simulink library "LIB_CycleControl"  (R2018b)
settings: Solver=VariableStepAuto  StartTime=0.0  StopTime=10.0  RelTol=1e-3
undefined symbols (not defined in the file or in its folder): eActuators, eRespiratorStates, NActuatorActive, nBlowerCmdInit, nBlowerCmdMax, nBlowerCmdMin, nBlowerDecHigh, nBlowerDecMedium, nBlowerIncHigh, nBlowerIncLow, nBlowerIncMedium, NBlowerSpeedIncCorrectionGain, NBlowerValveDerivativeGain, NBlowerValveIntegralGain, NBlowerValveIntegralHighGain, NBlowerValvePropGain, NCyclePerMinMax, NCyclePerMinMin, NMaxPressureSample, NPatientValveDerivativeGain, NPatientValveIntegralGain, NPatientValveIntegralHighGain, NPatientValvePropGain, pBlowerValveOutletOffset, pDiffMaxThdForPlateauPlausibility, pDiffThdForBlowerValveControlActivation, pDiffThdForPatientValveControlActivation, pErrorPlausibilityThd, pErrorThdForHighBlowerDec, pStaticErrorThdForHighBlowerInc, rPIDIntegralMaxTermForBlowerValve, rPIDIntegralMaxTermForPatientValve, rPIDIntegralMinTermForBlowerValve, rPIDIntegralMinTermForPatientValve, tBlowerValveOpen, tDelayBeforeRespiratorCycleStart, tDelayForRespiratorStop, tPatientValveOpen, tPhase1Ofs, tStopInhalationPhase1Min
libraries: simulink x62, simulink_need_slupdate x4, simulink_extras x3
(part 3 of 4)

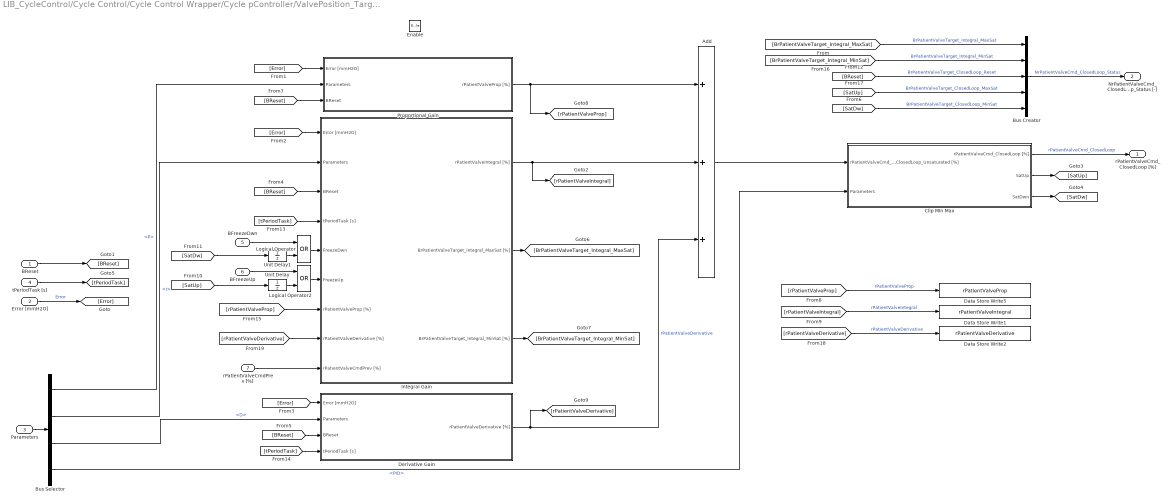
== system LIB_CycleControl/Cycle Control/Cycle Control Wrapper/Cycle pController/ValvePosition_Target/Exhalation/Patient Valve Control/PID Patient Valve ==
  BReset : Inport
  Error [mmH2O] : Inport  Port=2
  Parameters : Inport  Port=3
  tPeriodTask [s] : Inport  Port=4
  BFreezeDwn : Inport  Port=5
  BFreezeUp : Inport  Port=6
  rPatientValveCmdPrev [%] : Inport  Port=7
  Enable : EnablePort
  Add : Sum  Inputs=+++
  Bus Creator : BusCreator  Inputs=5
  Bus Selector : BusSelector  OutputSignals=P,I,D,PID
  Clip MIn Max : Subsystem
  Data Store Write1 : DataStoreWrite  DataStoreName=rPatientValveIntegral
  Data Store Write2 : DataStoreWrite  DataStoreName=rPatientValveDerivative
  Data Store Write5 : DataStoreWrite  DataStoreName=rPatientValveProp
  Derivative Gain : Subsystem
  Integral Gain : Subsystem
  Logical Operator : Logic  Operator=OR  AllPortsSameDT=off  OutDataTypeStr=boolean
  Logical Operator2 : Logic  Operator=OR  AllPortsSameDT=off  OutDataTypeStr=boolean
  Proportional Gain : Subsystem
  Unit Delay : UnitDelay  SampleTime=-1
  Unit Delay1 : UnitDelay  SampleTime=-1
  rPatientValveCmd_ClosedLoop [%] : Outport
  NrPatientValveCmd_ClosedLoop_Status [-] : Outport  Port=2
  wires:
  [rPatientValveDerivative] -> Data Store Write2/1  "rPatientValveDerivative"
  [rPatientValveIntegral] -> Data Store Write1/1  "rPatientValveIntegral"
  [rPatientValveProp] -> Data Store Write5/1  "rPatientValveProp"
  [BReset] -> Integral Gain/3(BReset)
  [rPatientValveDerivative] -> Integral Gain/8(rPatientValveDerivative [%])
  [rPatientValveProp] -> Integral Gain/7(rPatientValveProp [%])
  rPatientValveCmdPrev [%]/1 -> Integral Gain/9(rPatientValveCmdPrev [%])
  BReset/1 -> [BReset]
  [BReset] -> Derivative Gain/3(BReset)
  [BReset] -> Proportional Gain/3(BReset)
  [Error] -> Derivative Gain/1(Error [mmH2O])
  [Error] -> Integral Gain/1(Error [mmH2O])
  [Error] -> Proportional Gain/1(Error [mmH2O])
  Error [mmH2O]/1 -> [Error]  "Error"
  Clip MIn Max/1(rPatientValveCmd_ClosedLoop [%]) -> rPatientValveCmd_ClosedLoop [%]/1  "rPatientValveCmd_ClosedLoop"
  Bus Selector/4 -> Clip MIn Max/2(Parameters)  "<PID>"
  Add/1 -> Clip MIn Max/1(rPatientValveCmd_ClosedLoop_Unsaturated [%])
  Integral Gain/1(rPatientValveIntegral [%]) -> Add/2, [rPatientValveIntegral]
  Bus Selector/3 -> Derivative Gain/2(Parameters)  "<D>"
  Bus Selector/2 -> Integral Gain/2(Parameters)  "<I>"
  Bus Selector/1 -> Proportional Gain/2(Parameters)  "<P>"
  Parameters/1 -> Bus Selector/1
  [tPeriodTask] -> Integral Gain/4(tPeriodTask [s])
  Clip MIn Max/2(SatUp) -> [SatUp]
  Clip MIn Max/3(SatDwn) -> [SatDw]
  Logical Operator/1 -> Integral Gain/5(FreezeDwn)
  [SatDw] -> Unit Delay1/1
  BFreezeDwn/1 -> Logical Operator/1
  Logical Operator2/1 -> Integral Gain/6(FreezeUp)
  BFreezeUp/1 -> Logical Operator2/1
  [SatUp] -> Unit Delay/1
  Unit Delay/1 -> Logical Operator2/2
  Unit Delay1/1 -> Logical Operator/2
  tPeriodTask [s]/1 -> [tPeriodTask]
  [tPeriodTask] -> Derivative Gain/4(tPeriodTask [s])
  Integral Gain/3(BrPatientValveTarget_Integral_MinSat [%]) -> [BrPatientValveTarget_Integral_MinSat]
  Integral Gain/2(BrPatientValveTarget_Integral_MaxSat [%]) -> [BrPatientValveTarget_Integral_MaxSat]
  Bus Creator/1 -> NrPatientValveCmd_ClosedLoop_Status [-]/1  "NrPatientValveCmd_ClosedLoop_Status"
  Derivative Gain/1(rPatientValveDerivative [%]) -> Add/3, [rPatientValveDerivative]  "rPatientValveDerivative"
  Proportional Gain/1(rPatientValveProp [%]) -> Add/1, [rPatientValveProp]
  [BrPatientValveTarget_Integral_MaxSat] -> Bus Creator/1  "BrPatientValveTarget_Integral_MaxSat"
  [BrPatientValveTarget_Integral_MinSat] -> Bus Creator/2  "BrPatientValveTarget_Integral_MinSat"
  [BReset] -> Bus Creator/3  "BrPatientValveTarget_ClosedLoop_Reset"
  [SatUp] -> Bus Creator/4  "BrPatientValveTarget_ClosedLoop_MaxSat"
  [SatDw] -> Bus Creator/5  "BrPatientValveTarget_ClosedLoop_MinSat"

== system LIB_CycleControl/Cycle Control/Cycle Control Wrapper/Cycle pController/ValvePosition_Target/Exhalation/Patient Valve Control/Parameters ==
  note: 1/(2*Pi*Tau)
  Error [mmH2O] : Inport
  pBlowerValveOutletTarget [mmH2O] : Inport  Port=2
  Enable : EnablePort
  Bus Creator : BusCreator  Inputs=3
  Bus Creator1 : BusCreator  Inputs=3
  Bus Creator2 : BusCreator  Inputs=5
  Bus Creator3 : BusCreator  Inputs=5
  Bus Creator4 : BusCreator  Inputs='PidMax','PidMin'
  Constant1 : Constant  OutDataTypeStr=boolean
  Constant10 : Constant  Value=0  OutDataTypeStr=single
  Constant2 : Constant  Value=1/(2*pi*0.1)  OutDataTypeStr=single
  Constant25 : Constant  Value=100  OutDataTypeStr=single
  Constant26 : Constant  Value=-100  OutDataTypeStr=single
  Constant5 : Constant  Value=0  OutDataTypeStr=boolean
  Constant6 : Constant  Value=10  OutDataTypeStr=single
  Constant7 : Constant  Value=-10  OutDataTypeStr=single
  Constant9 : Constant  Value=100  OutDataTypeStr=single
  Gain PID Elaboration : Subsystem
  Parameters : Outport
  wires:
  pBlowerValveOutletTarget [mmH2O]/1 -> Gain PID Elaboration/2(pBlowerValveOutletTarget [mmH2O])
  Constant1/1 -> Bus Creator3/5  "Enable"
  Error [mmH2O]/1 -> Gain PID Elaboration/1(Error [mmH2O])
  Gain PID Elaboration/5(rPatientValveDerivativeGain [%/mmH2O]) -> Bus Creator2/5  "Gain"
  Constant2/1 -> Bus Creator2/4  "Freq"
  Constant5/1 -> Bus Creator2/3  "Enable"
  Constant7/1 -> Bus Creator2/2  "Min-"
  Constant6/1 -> Bus Creator2/1  "Max+"
  Constant25/1 -> Bus Creator/1  "Sat+"
  Constant26/1 -> Bus Creator/2  "Sat-"
  Gain PID Elaboration/2(rPIDIntegralMaxTermForBlowerValve [%]) -> Bus Creator1/1  "Max+"
  Gain PID Elaboration/3(rPIDIntegralMinTermForBlowerValve [%]) -> Bus Creator1/2  "Min-"
  Constant9/1 -> Bus Creator4/1  "PidMax"
  Constant10/1 -> Bus Creator4/2  "PidMin"
  Bus Creator3/1 -> Parameters/1
  Gain PID Elaboration/4(rPatientValveIntegralGain [%/mmH2O]) -> Bus Creator1/3  "Gain"
  Gain PID Elaboration/1(rPatientValveProportionalGain [%/mmH2O]) -> Bus Creator/3  "Gain"
  Bus Creator/1 -> Bus Creator3/1  "P"
  Bus Creator1/1 -> Bus Creator3/2  "I"
  Bus Creator2/1 -> Bus Creator3/3  "D"
  Bus Creator4/1 -> Bus Creator3/4  "PID"

== system LIB_CycleControl/Cycle Control/Cycle Control Wrapper/Cycle pController/ValvePosition_Target/Inhalation/Blower Valve Control/OL ==
  tPeriodTask [s] : Inport
  BExternalInit [-] : Inport  Port=2
  rBlowerValveCmdPrev [%] : Inport  Port=3
  Enable : EnablePort
  Constant1 : Constant  Value=tBlowerValveOpen  OutDataTypeStr=single
  Constant2 : Constant  Value=100  OutDataTypeStr=single
  Gain : Gain  Gain=-1
  Product : Product  Inputs=*/
  Product1 : Product  Inputs=*/
  Rate Lmiter : Subsystem  mask(Rate Limiter Dynamic){}
      mask help: Simulink:masks:RateLimiterDynamic_MD
  Switch3 : Switch  Criteria=u2 ~= 0
      settings: AttributesFormatString=%<Criteria>
  Unit Delay1 : UnitDelay  SampleTime=-1
  rBlowerValveOLCmd [%] : Outport
  wires:
  Constant1/1 -> Product1/2, Product/2
  Unit Delay1/1 -> Switch3/3
  tPeriodTask [s]/1 -> Rate Lmiter/1(tPeriodTask [s])
  BExternalInit [-]/1 -> Switch3/2
  Product1/1 -> Rate Lmiter/4(lo)
  Product/1 -> Rate Lmiter/2(up)
  rBlowerValveCmdPrev [%]/1 -> Switch3/1
  Switch3/1 -> Rate Lmiter/5(Y(k-1))
  Rate Lmiter/1(Y(k)) -> Unit Delay1/1, rBlowerValveOLCmd [%]/1
  Constant2/1 -> Gain/1, Product/1, Rate Lmiter/3(u)
  Gain/1 -> Product1/1

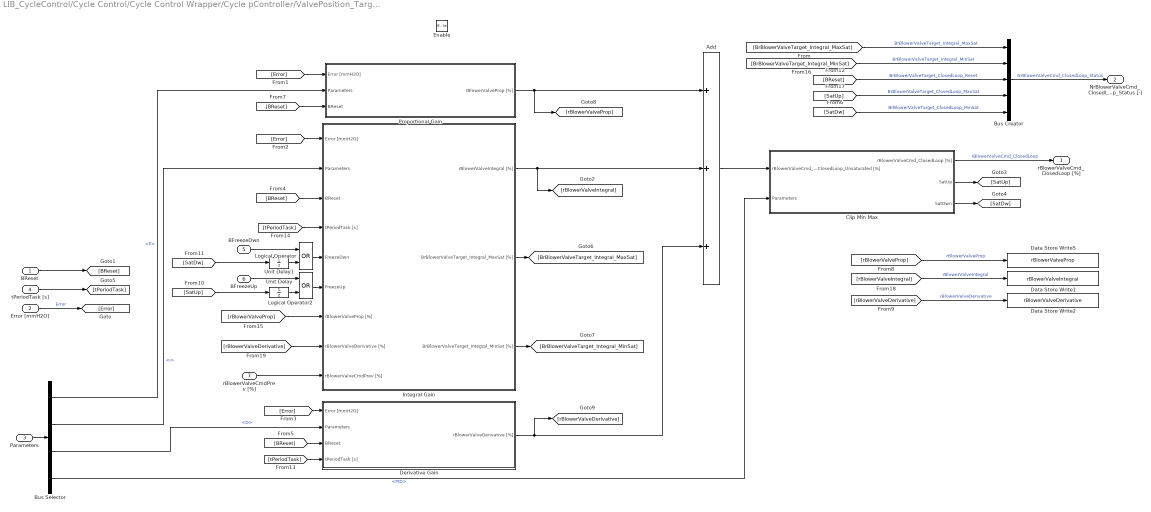
== system LIB_CycleControl/Cycle Control/Cycle Control Wrapper/Cycle pController/ValvePosition_Target/Inhalation/Blower Valve Control/PID Blower Valve ==
  BReset : Inport
  Error [mmH2O] : Inport  Port=2
  Parameters : Inport  Port=3
  tPeriodTask [s] : Inport  Port=4
  BFreezeDwn : Inport  Port=5
  BFreezeUp : Inport  Port=6
  rBlowerValveCmdPrev [%] : Inport  Port=7
  Enable : EnablePort
  Add : Sum  Inputs=+++
  Bus Creator : BusCreator  Inputs=5
  Bus Selector : BusSelector  OutputSignals=P,I,D,PID
  Clip MIn Max : Subsystem
  Data Store Write1 : DataStoreWrite  DataStoreName=rBlowerValveIntegral
  Data Store Write2 : DataStoreWrite  DataStoreName=rBlowerValveDerivative
  Data Store Write5 : DataStoreWrite  DataStoreName=rBlowerValveProp
  Derivative Gain : Subsystem
  Integral Gain : Subsystem
  Logical Operator : Logic  Operator=OR  AllPortsSameDT=off  OutDataTypeStr=boolean
  Logical Operator2 : Logic  Operator=OR  AllPortsSameDT=off  OutDataTypeStr=boolean
  Proportional Gain : Subsystem
  Unit Delay : UnitDelay  SampleTime=-1
  Unit Delay1 : UnitDelay  SampleTime=-1
  rBlowerValveCmd_ClosedLoop [%] : Outport
  NrBlowerValveCmd_ClosedLoop_Status [-] : Outport  Port=2
  wires:
  [rBlowerValveDerivative] -> Data Store Write2/1  "rBlowerValveDerivative"
  [rBlowerValveIntegral] -> Data Store Write1/1  "rBlowerValveIntegral"
  [rBlowerValveProp] -> Data Store Write5/1  "rBlowerValveProp"
  [BReset] -> Integral Gain/3(BReset)
  [rBlowerValveDerivative] -> Integral Gain/8(rBlowerValveDerivative [%])
  [rBlowerValveProp] -> Integral Gain/7(rBlowerValveProp [%])
  rBlowerValveCmdPrev [%]/1 -> Integral Gain/9(rBlowerValveCmdPrev [%])
  BReset/1 -> [BReset]
  [BReset] -> Derivative Gain/3(BReset)
  [BReset] -> Proportional Gain/3(BReset)
  [Error] -> Derivative Gain/1(Error [mmH2O])
  [Error] -> Integral Gain/1(Error [mmH2O])
  [Error] -> Proportional Gain/1(Error [mmH2O])
  Error [mmH2O]/1 -> [Error]  "Error"
  Clip MIn Max/1(rBlowerValveCmd_ClosedLoop [%]) -> rBlowerValveCmd_ClosedLoop [%]/1  "rBlowerValveCmd_ClosedLoop"
  Bus Selector/4 -> Clip MIn Max/2(Parameters)  "<PID>"
  Add/1 -> Clip MIn Max/1(rBlowerValveCmd_ClosedLoop_Unsaturated [%])
  Integral Gain/1(rBlowerValveIntegral [%]) -> Add/2, [rBlowerValveIntegral]
  Bus Selector/3 -> Derivative Gain/2(Parameters)  "<D>"
  Bus Selector/2 -> Integral Gain/2(Parameters)  "<I>"
  Bus Selector/1 -> Proportional Gain/2(Parameters)  "<P>"
  Parameters/1 -> Bus Selector/1
  [tPeriodTask] -> Integral Gain/4(tPeriodTask [s])
  Clip MIn Max/2(SatUp) -> [SatUp]
  Clip MIn Max/3(SatDwn) -> [SatDw]
  Logical Operator/1 -> Integral Gain/5(FreezeDwn)
  [SatDw] -> Unit Delay1/1
  BFreezeDwn/1 -> Logical Operator/1
  Logical Operator2/1 -> Integral Gain/6(FreezeUp)
  BFreezeUp/1 -> Logical Operator2/1
  [SatUp] -> Unit Delay/1
  Unit Delay/1 -> Logical Operator2/2
  Unit Delay1/1 -> Logical Operator/2
  tPeriodTask [s]/1 -> [tPeriodTask]
  [tPeriodTask] -> Derivative Gain/4(tPeriodTask [s])
  Integral Gain/3(BrBlowerValveTarget_Integral_MinSat [%]) -> [BrBlowerValveTarget_Integral_MinSat]
  Integral Gain/2(BrBlowerValveTarget_Integral_MaxSat [%]) -> [BrBlowerValveTarget_Integral_MaxSat]
  Bus Creator/1 -> NrBlowerValveCmd_ClosedLoop_Status [-]/1  "NrBlowerValveCmd_ClosedLoop_Status"
  Derivative Gain/1(rBlowerValveDerivative [%]) -> Add/3, [rBlowerValveDerivative]
  Proportional Gain/1(rBlowerValveProp [%]) -> Add/1, [rBlowerValveProp]
  [BrBlowerValveTarget_Integral_MaxSat] -> Bus Creator/1  "BrBlowerValveTarget_Integral_MaxSat"
  [BrBlowerValveTarget_Integral_MinSat] -> Bus Creator/2  "BrBlowerValveTarget_Integral_MinSat"
  [BReset] -> Bus Creator/3  "BrBlowerValveTarget_ClosedLoop_Reset"
  [SatUp] -> Bus Creator/4  "BrBlowerValveTarget_ClosedLoop_MaxSat"
  [SatDw] -> Bus Creator/5  "BrBlowerValveTarget_ClosedLoop_MinSat"

== system LIB_CycleControl/Cycle Control/Cycle Control Wrapper/Cycle pController/ValvePosition_Target/Inhalation/Blower Valve Control/Parameters ==
  note: 1/(2*Pi*Tau)
  Error : Inport
  Enable : EnablePort
  Bus Creator : BusCreator  Inputs=3
  Bus Creator1 : BusCreator  Inputs=3
  Bus Creator2 : BusCreator  Inputs=5
  Bus Creator3 : BusCreator  Inputs=5
  Bus Creator4 : BusCreator  Inputs='PidMax','PidMin'
  Constant1 : Constant  OutDataTypeStr=boolean
  Constant10 : Constant  Value=0  OutDataTypeStr=single
  Constant2 : Constant  Value=1/(2*pi*0.1)  OutDataTypeStr=single
  Constant25 : Constant  Value=100  OutDataTypeStr=single
  Constant26 : Constant  Value=-100  OutDataTypeStr=single
  Constant5 : Constant  Value=0  OutDataTypeStr=boolean
  Constant6 : Constant  Value=10  OutDataTypeStr=single
  Constant7 : Constant  Value=-10  OutDataTypeStr=single
  Constant9 : Constant  Value=100  OutDataTypeStr=single
  Gain PID Elaboration : Subsystem
  Parameters : Outport
  wires:
  Constant1/1 -> Bus Creator3/5  "Enable"
  Gain PID Elaboration/5(rBlowerValveDerivativeGain [%/mmH2O]) -> Bus Creator2/5  "Gain"
  Constant2/1 -> Bus Creator2/4  "Freq"
  Constant5/1 -> Bus Creator2/3  "Enable"
  Constant7/1 -> Bus Creator2/2  "Min-"
  Constant6/1 -> Bus Creator2/1  "Max+"
  Constant25/1 -> Bus Creator/1  "Sat+"
  Constant26/1 -> Bus Creator/2  "Sat-"
  Gain PID Elaboration/2(rPIDIntegralMaxTermForBlowerValve [%]) -> Bus Creator1/1  "Max+"
  Gain PID Elaboration/3(rPIDIntegralMinTermForBlowerValve [%]) -> Bus Creator1/2  "Min-"
  Constant9/1 -> Bus Creator4/1  "PidMax"
  Constant10/1 -> Bus Creator4/2  "PidMin"
  Bus Creator3/1 -> Parameters/1
  Gain PID Elaboration/4(rBlowerValveIntegralGain [%/mmH2O]) -> Bus Creator1/3  "Gain"
  Gain PID Elaboration/1(rBlowerValveProportionalGain [%/mmH2O]) -> Bus Creator/3  "Gain"
  Bus Creator/1 -> Bus Creator3/1  "P"
  Bus Creator1/1 -> Bus Creator3/2  "I"
  Bus Creator2/1 -> Bus Creator3/3  "D"
  Bus Creator4/1 -> Bus Creator3/4  "PID"
  Error/1 -> Gain PID Elaboration/1(Error)

== system LIB_CycleControl/Cycle Control/Cycle Control Wrapper/Cycle pController/ValvePosition_Target/Exhalation/Patient Valve Control/OL1/Rate Lmiter ==
  note: Y(k)
  tPeriodTask [s] : Inport
  up : Inport  Port=2
  u : Inport  Port=3
  lo : Inport  Port=4
  Y(k-1) : Inport  Port=5
  Difference Inputs1 : Sum  Description=Add in CPU  DisableCoverage=on  Inputs=+-  OutDataTypeStr=Inherit: Inherit via back propagation
  Difference Inputs2 : Sum  Description=Add in CPU  OutDataTypeStr=Inherit: Inherit via back propagation
  Saturation Dynamic : simulink/Discontinuities/Saturation Dynamic  OutMin=[]  OutMax=[]  OutDataTypeStr=Inherit: Same as second input  OutDataType=fixdt(1, 16)  OutScaling=2^-10  DoSatur=off
  delta fall limit : Product  DisableCoverage=on  Inputs=**  OutDataTypeStr=Inherit: Inherit via back propagation  SaturateOnIntegerOverflow=on
  delta rise limit : Product  DisableCoverage=on  Inputs=**  OutDataTypeStr=Inherit: Inherit via back propagation  SaturateOnIntegerOverflow=on
  Y(k) : Outport
  wires:
  Y(k-1)/1 -> Difference Inputs1/2, Difference Inputs2/2
  lo/1 -> delta fall limit/1
  u/1 -> Difference Inputs1/1
  up/1 -> delta rise limit/1
  Difference Inputs2/1 -> Y(k)/1
  delta fall limit/1 -> Saturation Dynamic/3
  delta rise limit/1 -> Saturation Dynamic/1
  Saturation Dynamic/1 -> Difference Inputs2/1
  Difference Inputs1/1 -> Saturation Dynamic/2  "( U(k) - Y(k-1) )"
  tPeriodTask [s]/1 -> delta rise limit/2, delta fall limit/2

== system LIB_CycleControl/Cycle Control/Cycle Control Wrapper/Cycle pController/ValvePosition_Target/Exhalation/Patient Valve Control/PID Patient Valve/Clip MIn Max ==
  rPatientValveCmd_ClosedLoop_Unsaturated [%] : Inport
  Parameters : Inport  Port=2
  Bus Selector : BusSelector  OutputSignals=PidMax,PidMin
  Clip1 : Subsystem  mask(PT Common Clip){}
      mask help: Input is clipped between the upper and lower limits.
      mask Help: helpview(fullfile(ptcommonroot,'help', 'clip.htm'))
  rPatientValveCmd_ClosedLoop [%] : Outport
  SatUp : Outport  Port=2
  SatDwn : Outport  Port=3
  wires:
  Clip1/2(Out) -> rPatientValveCmd_ClosedLoop [%]/1
  rPatientValveCmd_ClosedLoop_Unsaturated [%]/1 -> Clip1/2(In)
  Bus Selector/1 -> Clip1/1(Upper)  "<PidMax>"
  Parameters/1 -> Bus Selector/1
  Bus Selector/2 -> Clip1/3(Lower)  "<PidMin>"
  Clip1/1(SatUp) -> SatUp/1
  Clip1/3(SatDwn) -> SatDwn/1

== system LIB_CycleControl/Cycle Control/Cycle Control Wrapper/Cycle pController/ValvePosition_Target/Exhalation/Patient Valve Control/PID Patient Valve/Derivative Gain ==
  note: Derivative
  Error [mmH2O] : Inport
  Parameters : Inport  Port=2
  BReset : Inport  Port=3
  tPeriodTask [s] : Inport  Port=4
  Bus Selector : BusSelector  OutputSignals=Enable,Gain,Max+,Min-,Freq
  Compute Derivative : Subsystem
  rPatientValveDerivative [%] : Outport
  wires:
  [BReset] -> Compute Derivative/5(BReset)
  Bus Selector/1 -> Compute Derivative/Enable  "<Enable>"
  Bus Selector/5 -> Compute Derivative/4(Freq)  "<Freq>"
  Bus Selector/4 -> Compute Derivative/3(Min-)  "<Min->"
  Bus Selector/3 -> Compute Derivative/2(Max+)  "<Max+>"
  Bus Selector/2 -> Compute Derivative/1(Gain)  "<Gain>"
  tPeriodTask [s]/1 -> Compute Derivative/7(tPeriodTask [s])
  Error [mmH2O]/1 -> Compute Derivative/6(Error [mmH2O])
  BReset/1 -> [BReset]
  Parameters/1 -> Bus Selector/1
  Compute Derivative/1(rPatientValveDerivative [%]) -> rPatientValveDerivative [%]/1

== system LIB_CycleControl/Cycle Control/Cycle Control Wrapper/Cycle pController/ValvePosition_Target/Exhalation/Patient Valve Control/PID Patient Valve/Integral Gain ==
  Error [mmH2O] : Inport
  Parameters : Inport  Port=2
  BReset : Inport  Port=3
  tPeriodTask [s] : Inport  Port=4
  FreezeDwn : Inport  Port=5
  FreezeUp : Inport  Port=6
  rPatientValveProp [%] : Inport  Port=7
  rPatientValveDerivative [%] : Inport  Port=8
  rPatientValveCmdPrev [%] : Inport  Port=9
  Bus Selector : BusSelector  OutputSignals=Gain,Max+,Min-
  Clip : Subsystem  mask(PT Common Clip){}
      mask help: Input is clipped between the upper and lower limits.
      mask Help: helpview(fullfile(ptcommonroot,'help', 'clip.htm'))
  Init : Subsystem
  Logical Operator : Logic  AllPortsSameDT=off  OutDataTypeStr=boolean
  Logical Operator2 : Logic  Operator=NOT  AllPortsSameDT=off  OutDataTypeStr=boolean
  Logical Operator3 : Logic  AllPortsSameDT=off  OutDataTypeStr=boolean
  Logical Operator4 : Logic  Operator=NOT  AllPortsSameDT=off  OutDataTypeStr=boolean
  Product1 : Product  Inputs=3  RndMeth=Zero
  Reset? : Switch  Criteria=u2 ~= 0
  Sum1 : Sum  Inputs=|++
  Sum2 : Sum  Inputs=|++
  Unit Delay1 : UnitDelay  SampleTime=-1
  rPatientValveIntegral [%] : Outport
  BrPatientValveTarget_Integral_MaxSat [%] : Outport  Port=2
  BrPatientValveTarget_Integral_MinSat [%] : Outport  Port=3
  wires:
  Bus Selector/1 -> Product1/3  "<Gain>"
  Sum2/1 -> Reset?/1
  Init/1(Init) -> Sum2/1
  Unit Delay1/1 -> Sum1/2
  [BReset] -> Init/Enable
  BReset/1 -> [BReset]
  rPatientValveProp [%]/1 -> Init/3(rPatientValveProp [%])
  rPatientValveDerivative [%]/1 -> Init/2(rPatientValveDerivative [%])
  rPatientValveCmdPrev [%]/1 -> Init/1(rPatientValveCmdPrev [%])
  Clip/2(Out) -> Unit Delay1/1, rPatientValveIntegral [%]/1  "Error"
  Sum1/1 -> Reset?/3
  Reset?/1 -> Clip/3(In)
  Error [mmH2O]/1 -> Product1/1  "Error"
  Product1/1 -> Sum1/1, Sum2/2  "Gain*Error"
  Parameters/1 -> Bus Selector/1
  tPeriodTask [s]/1 -> Product1/2
  FreezeDwn/1 -> Logical Operator3/1
  FreezeUp/1 -> Logical Operator/1
  Clip/1(SatUp) -> BrPatientValveTarget_Integral_MaxSat [%]/1
  Clip/3(SatDwn) -> BrPatientValveTarget_Integral_MinSat [%]/1
  Bus Selector/3 -> [SatDwn]  "<Min->"
  Bus Selector/2 -> [SatUp]  "<Max+>"
  [SatUp] -> Clip/2(Upper)
  [SatDwn] -> Clip/4(Lower)
  Logical Operator/1 -> Clip/1(FreezeUp)
  Logical Operator2/1 -> Logical Operator/2
  Logical Operator3/1 -> Clip/5(FreezeDwn)
  Logical Operator4/1 -> Logical Operator3/2
  [BReset] -> Reset?/2, Logical Operator2/1, Logical Operator4/1

== system LIB_CycleControl/Cycle Control/Cycle Control Wrapper/Cycle pController/ValvePosition_Target/Exhalation/Patient Valve Control/PID Patient Valve/Proportional Gain ==
  Error [mmH2O] : Inport
  Parameters : Inport  Port=2
  BReset : Inport  Port=3
  Bus Selector : BusSelector  OutputSignals=Gain,Sat+,Sat-
  Clip : Subsystem  mask(PT Common Clip){}
      mask help: Input is clipped between the upper and lower limits.
      mask Help: helpview(fullfile(ptcommonroot,'help', 'clip.htm'))
  Constant : Constant  Value=0  OutDataTypeStr=single
  Product : Product  RndMeth=Zero
  Switch : Switch  Criteria=u2 ~= 0
  rPatientValveProp [%] : Outport
  wires:
  Parameters/1 -> Bus Selector/1
  Bus Selector/1 -> Product/1  "<Gain>"
  Switch/1 -> Product/2  "Error"
  BReset/1 -> Switch/2
  Constant/1 -> Switch/1
  Error [mmH2O]/1 -> Switch/3
  Bus Selector/2 -> Clip/1(Upper)  "<Sat+>"
  Bus Selector/3 -> Clip/3(Lower)  "<Sat->"
  Product/1 -> Clip/2(In)  "Gain*Error"
  Clip/1(Out) -> rPatientValveProp [%]/1

== system LIB_CycleControl/Cycle Control/Cycle Control Wrapper/Cycle pController/ValvePosition_Target/Exhalation/Patient Valve Control/Parameters/Gain PID Elaboration ==
  Error [mmH2O] : Inport
  pBlowerValveOutletTarget [mmH2O] : Inport  Port=2
  Compare To Zero : simulink/Logic and Bit Operations/Compare To Zero  relop=>  OutDataTypeStr=boolean
  Constant1 : Constant  Value=NPatientValveIntegralHighGain
  Constant28 : Constant  Value=NPatientValveIntegralGain
  Constant29 : Constant  Value=NPatientValveDerivativeGain
  Constant30 : Constant  Value=rPIDIntegralMaxTermForPatientValve
  Constant31 : Constant  Value=rPIDIntegralMinTermForPatientValve
  Constant32 : Constant  Value=NPatientValvePropGain
  Conv mmH2O to % : Gain  Gain=-100/1000
  Gain1 : Gain  Gain=-100/1000
  Gain2 : Gain  Gain=-100/1000
  NIntegralCorrectionPeep : Lookup_n-D  NumberOfTableDimensions=1  BreakpointsForDimension1=[0 50 100 150 200]  IndexSearchMethod=Linear search  BeginIndexSearchUsingPreviousIndexResult=on  Table=[1.5 1.5 1 0.5 0.5]  ExtrapMethod=Clip  UseLastTableValue=on  InternalRulePriority=Speed  RndMeth=Simplest  InputSameDT=on
  NPropCorrectionPeep : Lookup_n-D  NumberOfTableDimensions=1  BreakpointsForDimension1=[0 50 100 150 200]  IndexSearchMethod=Linear search  BeginIndexSearchUsingPreviousIndexResult=on  Table=[1 1 1 1 1]  ExtrapMethod=Clip  UseLastTableValue=on  InternalRulePriority=Speed  RndMeth=Simplest  InputSameDT=on
  Product : Product
  Product1 : Product
  Switch7 : Switch  Criteria=u2 ~= 0
      settings: AttributesFormatString=%<Criteria>
  rPatientValveProportionalGain [%/mmH2O] : Outport
  rPIDIntegralMaxTermForBlowerValve [%] : Outport  Port=2
  rPIDIntegralMinTermForBlowerValve [%] : Outport  Port=3
  rPatientValveIntegralGain [%/mmH2O] : Outport  Port=4
  rPatientValveDerivativeGain [%/mmH2O] : Outport  Port=5
  wires:
  Product1/1 -> Gain1/1
  NIntegralCorrectionPeep/1 -> Product1/1
  Switch7/1 -> Product1/2
  Error [mmH2O]/1 -> Compare To Zero/1
  Constant1/1 -> Switch7/1
  NPropCorrectionPeep/1 -> Product/2
  Constant32/1 -> Product/1
  Compare To Zero/1 -> Switch7/2
  Constant28/1 -> Switch7/3
  pBlowerValveOutletTarget [mmH2O]/1 -> NPropCorrectionPeep/1, NIntegralCorrectionPeep/1
  Constant31/1 -> rPIDIntegralMinTermForBlowerValve [%]/1
  Constant30/1 -> rPIDIntegralMaxTermForBlowerValve [%]/1
  Constant29/1 -> Gain2/1
  Product/1 -> Conv mmH2O to %/1
  Gain2/1 -> rPatientValveDerivativeGain [%/mmH2O]/1
  Conv mmH2O to %/1 -> rPatientValveProportionalGain [%/mmH2O]/1
  Gain1/1 -> rPatientValveIntegralGain [%/mmH2O]/1

== system LIB_CycleControl/Cycle Control/Cycle Control Wrapper/Cycle pController/ValvePosition_Target/Inhalation/Blower Valve Control/OL/Rate Lmiter ==
  note: Y(k)
  tPeriodTask [s] : Inport
  up : Inport  Port=2
  u : Inport  Port=3
  lo : Inport  Port=4
  Y(k-1) : Inport  Port=5
  Difference Inputs1 : Sum  Description=Add in CPU  DisableCoverage=on  Inputs=+-  OutDataTypeStr=Inherit: Inherit via back propagation
  Difference Inputs2 : Sum  Description=Add in CPU  OutDataTypeStr=Inherit: Inherit via back propagation
  Saturation Dynamic : simulink/Discontinuities/Saturation Dynamic  OutMin=[]  OutMax=[]  OutDataTypeStr=Inherit: Same as second input  OutDataType=fixdt(1, 16)  OutScaling=2^-10  DoSatur=off
  delta fall limit : Product  DisableCoverage=on  Inputs=**  OutDataTypeStr=Inherit: Inherit via back propagation  SaturateOnIntegerOverflow=on
  delta rise limit : Product  DisableCoverage=on  Inputs=**  OutDataTypeStr=Inherit: Inherit via back propagation  SaturateOnIntegerOverflow=on
  Y(k) : Outport
  wires:
  Y(k-1)/1 -> Difference Inputs1/2, Difference Inputs2/2
  lo/1 -> delta fall limit/1
  u/1 -> Difference Inputs1/1
  up/1 -> delta rise limit/1
  Difference Inputs2/1 -> Y(k)/1
  delta fall limit/1 -> Saturation Dynamic/3
  delta rise limit/1 -> Saturation Dynamic/1
  Saturation Dynamic/1 -> Difference Inputs2/1
  Difference Inputs1/1 -> Saturation Dynamic/2  "( U(k) - Y(k-1) )"
  tPeriodTask [s]/1 -> delta rise limit/2, delta fall limit/2

== system LIB_CycleControl/Cycle Control/Cycle Control Wrapper/Cycle pController/ValvePosition_Target/Inhalation/Blower Valve Control/PID Blower Valve/Clip MIn Max ==
  rBlowerValveCmd_ClosedLoop_Unsaturated [%] : Inport
  Parameters : Inport  Port=2
  Bus Selector : BusSelector  OutputSignals=PidMax,PidMin
  Clip1 : Subsystem  mask(PT Common Clip){}
      mask help: Input is clipped between the upper and lower limits.
      mask Help: helpview(fullfile(ptcommonroot,'help', 'clip.htm'))
  rBlowerValveCmd_ClosedLoop [%] : Outport
  SatUp : Outport  Port=2
  SatDwn : Outport  Port=3
  wires:
  Clip1/2(Out) -> rBlowerValveCmd_ClosedLoop [%]/1
  rBlowerValveCmd_ClosedLoop_Unsaturated [%]/1 -> Clip1/2(In)
  Bus Selector/1 -> Clip1/1(Upper)  "<PidMax>"
  Parameters/1 -> Bus Selector/1
  Bus Selector/2 -> Clip1/3(Lower)  "<PidMin>"
  Clip1/1(SatUp) -> SatUp/1
  Clip1/3(SatDwn) -> SatDwn/1

== system LIB_CycleControl/Cycle Control/Cycle Control Wrapper/Cycle pController/ValvePosition_Target/Inhalation/Blower Valve Control/PID Blower Valve/Derivative Gain ==
  note: Derivative
  Error [mmH2O] : Inport
  Parameters : Inport  Port=2
  BReset : Inport  Port=3
  tPeriodTask [s] : Inport  Port=4
  Bus Selector : BusSelector  OutputSignals=Enable,Gain,Max+,Min-,Freq
  Compute Derivative : Subsystem
  rBlowerValveDerivative [%] : Outport
  wires:
  [BReset] -> Compute Derivative/5(BReset)
  Bus Selector/1 -> Compute Derivative/Enable  "<Enable>"
  Bus Selector/5 -> Compute Derivative/4(Freq)  "<Freq>"
  Bus Selector/4 -> Compute Derivative/3(Min-)  "<Min->"
  Bus Selector/3 -> Compute Derivative/2(Max+)  "<Max+>"
  Bus Selector/2 -> Compute Derivative/1(Gain)  "<Gain>"
  tPeriodTask [s]/1 -> Compute Derivative/7(tPeriodTask [s])
  Error [mmH2O]/1 -> Compute Derivative/6(Error [mmH2O])
  BReset/1 -> [BReset]
  Parameters/1 -> Bus Selector/1
  Compute Derivative/1(rBlowerValveDerivative [%]) -> rBlowerValveDerivative [%]/1

== system LIB_CycleControl/Cycle Control/Cycle Control Wrapper/Cycle pController/ValvePosition_Target/Inhalation/Blower Valve Control/PID Blower Valve/Integral Gain ==
  Error [mmH2O] : Inport
  Parameters : Inport  Port=2
  BReset : Inport  Port=3
  tPeriodTask [s] : Inport  Port=4
  FreezeDwn : Inport  Port=5
  FreezeUp : Inport  Port=6
  rBlowerValveProp [%] : Inport  Port=7
  rBlowerValveDerivative [%] : Inport  Port=8
  rBlowerValveCmdPrev [%] : Inport  Port=9
  Bus Selector : BusSelector  OutputSignals=Gain,Max+,Min-
  Clip : Subsystem  mask(PT Common Clip){}
      mask help: Input is clipped between the upper and lower limits.
      mask Help: helpview(fullfile(ptcommonroot,'help', 'clip.htm'))
  Init : Subsystem
  Logical Operator : Logic  AllPortsSameDT=off  OutDataTypeStr=boolean
  Logical Operator2 : Logic  Operator=NOT  AllPortsSameDT=off  OutDataTypeStr=boolean
  Logical Operator3 : Logic  AllPortsSameDT=off  OutDataTypeStr=boolean
  Logical Operator4 : Logic  Operator=NOT  AllPortsSameDT=off  OutDataTypeStr=boolean
  Product1 : Product  Inputs=3  RndMeth=Zero
  Reset? : Switch  Criteria=u2 ~= 0
  Sum1 : Sum  Inputs=|++
  Sum2 : Sum  Inputs=|++
  Unit Delay1 : UnitDelay  SampleTime=-1
  rBlowerValveIntegral [%] : Outport
  BrBlowerValveTarget_Integral_MaxSat [%] : Outport  Port=2
  BrBlowerValveTarget_Integral_MinSat [%] : Outport  Port=3
  wires:
  Bus Selector/1 -> Product1/3  "<Gain>"
  Init/1(Init) -> Sum2/1
  Unit Delay1/1 -> Sum1/2
  Sum2/1 -> Reset?/1
  [BReset] -> Init/Enable
  BReset/1 -> [BReset]
  rBlowerValveProp [%]/1 -> Init/3(rBlowerValveProp [%])
  rBlowerValveDerivative [%]/1 -> Init/2(rBlowerValveDerivative [%])
  rBlowerValveCmdPrev [%]/1 -> Init/1(rBlowerValveCmdPrev [%])
  Clip/2(Out) -> Unit Delay1/1, rBlowerValveIntegral [%]/1  "Error"
  Sum1/1 -> Reset?/3
  Reset?/1 -> Clip/3(In)
  Error [mmH2O]/1 -> Product1/1  "Error"
  Product1/1 -> Sum1/1, Sum2/2  "Gain*Error"
  Parameters/1 -> Bus Selector/1
  tPeriodTask [s]/1 -> Product1/2
  FreezeDwn/1 -> Logical Operator3/1
  FreezeUp/1 -> Logical Operator/1
  Clip/1(SatUp) -> BrBlowerValveTarget_Integral_MaxSat [%]/1
  Clip/3(SatDwn) -> BrBlowerValveTarget_Integral_MinSat [%]/1
  Bus Selector/3 -> [SatDwn]  "<Min->"
  Bus Selector/2 -> [SatUp]  "<Max+>"
  [SatUp] -> Clip/2(Upper)
  [SatDwn] -> Clip/4(Lower)
  Logical Operator/1 -> Clip/1(FreezeUp)
  Logical Operator2/1 -> Logical Operator/2
  Logical Operator3/1 -> Clip/5(FreezeDwn)
  Logical Operator4/1 -> Logical Operator3/2
  [BReset] -> Reset?/2, Logical Operator2/1, Logical Operator4/1

== system LIB_CycleControl/Cycle Control/Cycle Control Wrapper/Cycle pController/ValvePosition_Target/Inhalation/Blower Valve Control/PID Blower Valve/Proportional Gain ==
  Error [mmH2O] : Inport
  Parameters : Inport  Port=2
  BReset : Inport  Port=3
  Bus Selector : BusSelector  OutputSignals=Gain,Sat+,Sat-
  Clip : Subsystem  mask(PT Common Clip){}
      mask help: Input is clipped between the upper and lower limits.
      mask Help: helpview(fullfile(ptcommonroot,'help', 'clip.htm'))
  Constant : Constant  Value=0  OutDataTypeStr=single
  Product : Product  RndMeth=Zero
  Switch : Switch  Criteria=u2 ~= 0
  rBlowerValveProp [%] : Outport
  wires:
  Parameters/1 -> Bus Selector/1
  Bus Selector/1 -> Product/1  "<Gain>"
  Switch/1 -> Product/2  "Error"
  BReset/1 -> Switch/2
  Constant/1 -> Switch/1
  Error [mmH2O]/1 -> Switch/3
  Bus Selector/2 -> Clip/1(Upper)  "<Sat+>"
  Bus Selector/3 -> Clip/3(Lower)  "<Sat->"
  Product/1 -> Clip/2(In)  "Gain*Error"
  Clip/1(Out) -> rBlowerValveProp [%]/1

== system LIB_CycleControl/Cycle Control/Cycle Control Wrapper/Cycle pController/ValvePosition_Target/Inhalation/Blower Valve Control/Parameters/Gain PID Elaboration ==
  Error : Inport
  Compare To Zero : simulink/Logic and Bit Operations/Compare To Zero  relop=>  OutDataTypeStr=boolean
  Constant1 : Constant  Value=NBlowerValveIntegralGain
  Constant23 : Constant  Value=NBlowerValveIntegralHighGain
  Constant24 : Constant  Value=NBlowerValveDerivativeGain
  Constant25 : Constant  Value=rPIDIntegralMaxTermForBlowerValve
  Constant26 : Constant  Value=rPIDIntegralMinTermForBlowerValve
  Constant27 : Constant  Value=NBlowerValvePropGain
  Conv mmH2O to % : Gain  Gain=100/1000
  Gain1 : Gain  Gain=100/1000
  Gain2 : Gain  Gain=100/1000
  Switch7 : Switch  Criteria=u2 ~= 0
      settings: AttributesFormatString=%<Criteria>
  rBlowerValveProportionalGain [%/mmH2O] : Outport
  rPIDIntegralMaxTermForBlowerValve [%] : Outport  Port=2
  rPIDIntegralMinTermForBlowerValve [%] : Outport  Port=3
  rBlowerValveIntegralGain [%/mmH2O] : Outport  Port=4
  rBlowerValveDerivativeGain [%/mmH2O] : Outport  Port=5
  wires:
  Constant23/1 -> Switch7/3
  Constant1/1 -> Switch7/1
  Error/1 -> Compare To Zero/1
  Compare To Zero/1 -> Switch7/2
  Constant25/1 -> rPIDIntegralMaxTermForBlowerValve [%]/1
  Constant26/1 -> rPIDIntegralMinTermForBlowerValve [%]/1
  Constant24/1 -> Conv mmH2O to %/1
  Conv mmH2O to %/1 -> rBlowerValveDerivativeGain [%/mmH2O]/1
  Gain1/1 -> rBlowerValveIntegralGain [%/mmH2O]/1
  Gain2/1 -> rBlowerValveProportionalGain [%/mmH2O]/1
  Constant27/1 -> Gain2/1
  Switch7/1 -> Gain1/1

== system LIB_CycleControl/Cycle Control/Cycle Control Wrapper/Cycle pController/ValvePosition_Target/Exhalation/Patient Valve Control/PID Patient Valve/Clip MIn Max/Clip1 ==
  note: 0,0
  note: 0,0
  note: 0,0
  Upper : Inport
  In : Inport  Port=2
  Lower : Inport  Port=3
  Logical Operator : Logic  Operator=NOT  AllPortsSameDT=off  OutDataTypeStr=boolean
  Relational Operator : RelationalOperator  Operator=<  RndMeth=Nearest  InputSameDT=on
  Relational Operator1 : RelationalOperator  Operator=>  RndMeth=Nearest  InputSameDT=on
  Switch : Switch  Threshold=1  SaturateOnIntegerOverflow=on  InputSameDT=on
  Switch1 : Switch  Threshold=1  SaturateOnIntegerOverflow=on  InputSameDT=on
  arround 0.001 : Subsystem
  SatUp : Outport
  Out : Outport  Port=2
  SatDwn : Outport  Port=3
  wires:
  Switch1/1 -> Out/1
  Relational Operator1/1 -> Switch1/2, Logical Operator/1
  Switch/1 -> Relational Operator1/1, Switch1/1
  Lower/1 -> Switch1/3, Relational Operator1/2
  Relational Operator/1 -> Switch/2, SatUp/1
  Upper/1 -> Relational Operator/1, Switch/1
  In/1 -> arround 0.001/1(In1)
  Logical Operator/1 -> SatDwn/1
  arround 0.001/1(Out1) -> Relational Operator/2, Switch/3

== system LIB_CycleControl/Cycle Control/Cycle Control Wrapper/Cycle pController/ValvePosition_Target/Exhalation/Patient Valve Control/PID Patient Valve/Derivative Gain/Compute Derivative ==
  note: dErr/dt
  Gain : Inport
  Max+ : Inport  Port=2
  Min- : Inport  Port=3
  Freq : Inport  Port=4
  BReset : Inport  Port=5
  Error [mmH2O] : Inport  Port=6
  tPeriodTask [s] : Inport  Port=7
  Enable : EnablePort
  Clip : Subsystem  mask(PT Common Clip){}
      mask help: Input is clipped between the upper and lower limits.
      mask Help: helpview(fullfile(ptcommonroot,'help', 'clip.htm'))
  Constant : Constant  Value=0  OutDataTypeStr=single
  Divide : Product  Inputs=*/
  Filtre_1er_ordre_Init : Subsystem  mask(FIRST ORDER FILTER INIT){TaskTime=SYNC, InType=Frequency}
      mask prompts: TaskTime "Task Execution Time"; InType "Filter Input Type :"
      mask help:
      | This block is a first-order filter with the following equation :
      | If f*Te< 0.5 with f=1(2*Pi*TAU)
      | y(k)=1/[1+Te/Tau]*y(k-1) + Te/Tau/[1+Te/Tau]*u(k).
      | Else y(k)=u(k)
      | In case of Reset, the output is initialized to INIT value.
      | In case of permanent reset, y(k)= INIT.
      mask init:
      | x=[-5:0.5:5];
      | y=1-exp(-(x+5)/1);
      | 
      | %get the mask level block path
      | blockPath=gcb;
      | 
      | %get the first inport and rename it depending on the value type selected by the user
      | Inports.Path=find_system(blockPath,'SearchDepth',1,'FollowLinks','on','regexp','on','LookUnderMasks','on','BlockType','Inport');
      | Inports.Handle=get_param(Inports.Path,'Handle');
      | Inports.Number=get_param(Inports.Path,'Port');
      | 
      | for i=1:1:length(Inports.Number)
      |     if strcmp(Inports.Number(i,1),'1')
      |         if strcmp(InType,'Tau')
      |             set_param(Inports.Handle{i,1},'Name','Tau [s]')
      |         else
      |             set_param(Inports.Handle{i,1},'Name','Frequency [Hz]')
      |         end
      |     end
      | end
      | 
      | Inports2.Path=find_system([blockPath '/Coefficients'],'SearchDepth',1,'FollowLinks','on','regexp','on','LookUnderMasks','on','BlockType','Inport');
      | Inports2.Handle=get_param(Inports2.Path,'Handle');
      | Inports2.Number=get_param(Inports2.Path,'Port');
      | 
      | for i=1:1:length(Inports2.Number)
      |     if strcmp(Inports2.Number(i,1),'1')
      |         if strcmp(InType,'Tau')
      |             set_param(Inports2.Handle{i,1},'Name','Tau [s]')
      |         else
      |             set_param(Inports2.Handle{i,1},'Name','Frequency [Hz]')
      |         end
      |     end
      | end
      | 
      | %find all constants
      | Constant.Path=find_system(blockPath,'SearchDepth',2,'FollowLinks','on','regexp','on','LookUnderMasks','on','BlockType','Constant');
      | Constant.Name=get_param(Constant.Path,'Name');
      | 
      | for i=1:1:length(Constant.Name(:,1))
      |     %set the constants for the selection Tau / frequency
      |     if strcmp(Constant.Name{i,1},'FilterInputTypeSelector')
      |         if strcmp(InType,'Frequency')
      |             set_param(Constant.Path{i,1},'Value','0')
      |         elseif strcmp(InType,'Tau')
      |             set_param(Constant.Path{i,1},'Value','1')
      |         end
      |     end
      | 
      |     %set the constants for the selection synchronous/asynchronous task time
      |     if strcmp(Constant.Name{i,1},'TaskTimeTypeSelector')
      |         if strcmp(TaskTime,'SYNC')
      |             set_param(Constant.Path{i,1},'Value','0')
      |         else
      |             set_param(Constant.Path{i,1},'Value','1')
      |         end
      |     end
      |     
      |     %set the constant for the task time
      |     if strcmp(Constant.Name{i,1},'Time') && ~strcmp(TaskTime,'SYNC')
      |         set_param(Constant.Path{i,1},'Value',num2str(str2double(regexprep(TaskTime,'ms',''))/1000))
      |     end
      | end
      mask Help:
      | This block is a first-order filter with the following equation :
      | If f*Te< 0.5 with f=1(2*Pi*TAU)
      | y(k)=1/[1+Te/Tau]*y(k-1) + Te/Tau/[1+Te/Tau]*u(k).
      | Else y(k)=u(k)
      | In case of Reset, the output is initialized to INIT value.
      | In case of permanent reset, y(k)= INIT.
      mask TypeOptions TaskTime: 1ms | 2ms | 5ms | 10ms | 20ms | 50ms | 100ms | 1000ms | SYNC
      mask TypeOptions InType: Tau | Frequency
      mask Display:
      | plot(x,y);
      | plot([min(x),max(x),NaN],[0,0,NaN]);
      | plot(min(-1,min(x)*1.5),min(-1,min(y)*1.5),max(1,max(x)*1.5),max(1,max(y)*1.5));
      | text(min(-0.9,min(x)*1.2),min(-0.9,min(y)*1.2),'First-Order Filter Init');
      | disp(['' TaskTime ''])% ] Cylinders \n Input Size : ' num2str(NTot)])
  Memory : Memory  InheritSampleTime=on
  Product : Product  RndMeth=Zero
  Sum : Sum  Inputs=|+-
  Switch : Switch  Criteria=u2 ~= 0
  rPatientValveDerivative [%] : Outport  OutputWhenDisabled=reset  InitialOutput=0
      settings: AttributesFormatString=%<OutputWhenDisabled>
  wires:
  [BReset] -> Switch/2
  [tPeriodTask] -> Filtre_1er_ordre_Init/5(PeriodTask [s])
  [tPeriodTask] -> Divide/2
  tPeriodTask [s]/1 -> [tPeriodTask]
  Gain/1 -> Product/2
  Switch/1 -> Product/1  "dErr/dt"
  Product/1 -> Clip/2(In)  "Gain*dErr/dt"
  Constant/1 -> Switch/1
  Sum/1 -> Divide/1
  Max+/1 -> Clip/1(Upper)
  Memory/1 -> Sum/2
  BReset/1 -> [BReset]
  Divide/1 -> Switch/3  "dErr_dT"
  Clip/1(Out) -> rPatientValveDerivative [%]/1
  Error [mmH2O]/1 -> Filtre_1er_ordre_Init/2(INPUT), Filtre_1er_ordre_Init/3(INIT)
  Min-/1 -> Clip/3(Lower)
  Filtre_1er_ordre_Init/1(OUTPUT) -> Sum/1, Memory/1
  Freq/1 -> Filtre_1er_ordre_Init/1(Frequency [Hz])
  [BReset] -> Filtre_1er_ordre_Init/4(RESET)

== system LIB_CycleControl/Cycle Control/Cycle Control Wrapper/Cycle pController/ValvePosition_Target/Exhalation/Patient Valve Control/PID Patient Valve/Integral Gain/Clip ==
  note: 0,0
  note: 0,0
  note: 0,0
  FreezeUp : Inport
  Upper : Inport  Port=2
  In : Inport  Port=3
  Lower : Inport  Port=4
  FreezeDwn : Inport  Port=5
  Logical Operator : Logic  Operator=NOT  AllPortsSameDT=off  OutDataTypeStr=boolean
  MinMax : MinMax  Inputs=2
  MinMax2 : MinMax  Function=max  Inputs=2
  Multiport Switch : MultiPortSwitch  DataPortOrder=Zero-based contiguous  Inputs=2  zeroidx=on
  Multiport Switch2 : MultiPortSwitch  DataPortOrder=Zero-based contiguous  Inputs=2  zeroidx=on
  Relational Operator : RelationalOperator  Operator=<  RndMeth=Nearest  InputSameDT=on
  Relational Operator1 : RelationalOperator  Operator=>  RndMeth=Nearest  InputSameDT=on
  Switch : Switch  Threshold=1  SaturateOnIntegerOverflow=on  InputSameDT=on
  Switch1 : Switch  Threshold=1  SaturateOnIntegerOverflow=on  InputSameDT=on
  Unit Delay External IC : simulink_need_slupdate/Unit Delay External IC  tsamp=-1
      settings: SourceProductName=Simulink  SourceProductBaseCode=SL
  Unit Delay External IC1 : simulink_need_slupdate/Unit Delay External IC  tsamp=-1
      settings: SourceProductName=Simulink  SourceProductBaseCode=SL
  arround 0.001 : Subsystem
  SatUp : Outport
  Out : Outport  Port=2
  SatDwn : Outport  Port=3
  wires:
  Switch1/1 -> Out/1, [Out]
  Relational Operator1/1 -> Switch1/2, Logical Operator/1
  Switch/1 -> Relational Operator1/1, Switch1/1
  Multiport Switch2/1 -> Switch1/3, Relational Operator1/2
  Relational Operator/1 -> Switch/2, SatUp/1
  In/1 -> arround 0.001/1(In1)
  Logical Operator/1 -> SatDwn/1
  Upper/1 -> Multiport Switch/2, MinMax/1, Unit Delay External IC/2
  Multiport Switch/1 -> Relational Operator/1, Switch/1
  FreezeUp/1 -> Multiport Switch/1
  MinMax/1 -> Multiport Switch/3
  Unit Delay External IC/1 -> MinMax/2
  Lower/1 -> MinMax2/1, Multiport Switch2/2, Unit Delay External IC1/2
  FreezeDwn/1 -> Multiport Switch2/1
  MinMax2/1 -> Multiport Switch2/3
  Unit Delay External IC1/1 -> MinMax2/2
  [Out] -> Unit Delay External IC/1
  [Out] -> Unit Delay External IC1/1
  arround 0.001/1(Out1) -> Relational Operator/2, Switch/3

== system LIB_CycleControl/Cycle Control/Cycle Control Wrapper/Cycle pController/ValvePosition_Target/Exhalation/Patient Valve Control/PID Patient Valve/Integral Gain/Init ==
  rPatientValveCmdPrev [%] : Inport
  rPatientValveDerivative [%] : Inport  Port=2
  rPatientValveProp [%] : Inport  Port=3
  Enable : EnablePort
  Sum2 : Sum  Inputs=+--
  Init : Outport
  wires:
  rPatientValveDerivative [%]/1 -> Sum2/3
  Sum2/1 -> Init/1
  rPatientValveCmdPrev [%]/1 -> Sum2/1
  rPatientValveProp [%]/1 -> Sum2/2

== system LIB_CycleControl/Cycle Control/Cycle Control Wrapper/Cycle pController/ValvePosition_Target/Exhalation/Patient Valve Control/PID Patient Valve/Proportional Gain/Clip ==
  note: 0,0
  note: 0,0
  note: 0,0
  Upper : Inport
  In : Inport  Port=2
  Lower : Inport  Port=3
  Relational Operator : RelationalOperator  Operator=<  RndMeth=Nearest  InputSameDT=on
  Relational Operator1 : RelationalOperator  Operator=>  RndMeth=Nearest  InputSameDT=on
  Switch : Switch  Threshold=1  SaturateOnIntegerOverflow=on  InputSameDT=on
  Switch1 : Switch  Threshold=1  SaturateOnIntegerOverflow=on  InputSameDT=on
  Out : Outport
  wires:
  Switch1/1 -> Out/1
  Relational Operator1/1 -> Switch1/2
  Switch/1 -> Relational Operator1/1, Switch1/1
  Lower/1 -> Switch1/3, Relational Operator1/2
  Relational Operator/1 -> Switch/2
  Upper/1 -> Relational Operator/1, Switch/1
  In/1 -> Relational Operator/2, Switch/3

== system LIB_CycleControl/Cycle Control/Cycle Control Wrapper/Cycle pController/ValvePosition_Target/Inhalation/Blower Valve Control/PID Blower Valve/Clip MIn Max/Clip1 ==
  note: 0,0
  note: 0,0
  note: 0,0
  Upper : Inport
  In : Inport  Port=2
  Lower : Inport  Port=3
  Logical Operator : Logic  Operator=NOT  AllPortsSameDT=off  OutDataTypeStr=boolean
  Relational Operator : RelationalOperator  Operator=<  RndMeth=Nearest  InputSameDT=on
  Relational Operator1 : RelationalOperator  Operator=>  RndMeth=Nearest  InputSameDT=on
  Switch : Switch  Threshold=1  SaturateOnIntegerOverflow=on  InputSameDT=on
  Switch1 : Switch  Threshold=1  SaturateOnIntegerOverflow=on  InputSameDT=on
  arround 0.001 : Subsystem
  SatUp : Outport
  Out : Outport  Port=2
  SatDwn : Outport  Port=3
  wires:
  Switch1/1 -> Out/1
  Relational Operator1/1 -> Switch1/2, Logical Operator/1
  Switch/1 -> Relational Operator1/1, Switch1/1
  Lower/1 -> Switch1/3, Relational Operator1/2
  Relational Operator/1 -> Switch/2, SatUp/1
  Upper/1 -> Relational Operator/1, Switch/1
  In/1 -> arround 0.001/1(In1)
  Logical Operator/1 -> SatDwn/1
  arround 0.001/1(Out1) -> Relational Operator/2, Switch/3

== system LIB_CycleControl/Cycle Control/Cycle Control Wrapper/Cycle pController/ValvePosition_Target/Inhalation/Blower Valve Control/PID Blower Valve/Derivative Gain/Compute Derivative ==
  Gain : Inport
  Max+ : Inport  Port=2
  Min- : Inport  Port=3
  Freq : Inport  Port=4
  BReset : Inport  Port=5
  Error [mmH2O] : Inport  Port=6
  tPeriodTask [s] : Inport  Port=7
  Enable : EnablePort
  Clip : Subsystem  mask(PT Common Clip){}
      mask help: Input is clipped between the upper and lower limits.
      mask Help: helpview(fullfile(ptcommonroot,'help', 'clip.htm'))
  Constant : Constant  Value=0  OutDataTypeStr=single
  Divide : Product  Inputs=*/
  Filtre_1er_ordre_Init : Subsystem  mask(FIRST ORDER FILTER INIT){TaskTime=SYNC, InType=Frequency}
      mask prompts: TaskTime "Task Execution Time"; InType "Filter Input Type :"
      mask help:
      | This block is a first-order filter with the following equation :
      | If f*Te< 0.5 with f=1(2*Pi*TAU)
      | y(k)=1/[1+Te/Tau]*y(k-1) + Te/Tau/[1+Te/Tau]*u(k).
      | Else y(k)=u(k)
      | In case of Reset, the output is initialized to INIT value.
      | In case of permanent reset, y(k)= INIT.
      mask init: same as LIB_CycleControl/Cycle Control/Cycle Control Wrapper/Cycle pController/ValvePosition_Target/Exhalation/Patient Valve Control/PID Patient Valve/Derivative Gain/Compute Derivative/Filtre_1er_ordre_Init
      mask Help:
      | This block is a first-order filter with the following equation :
      | If f*Te< 0.5 with f=1(2*Pi*TAU)
      | y(k)=1/[1+Te/Tau]*y(k-1) + Te/Tau/[1+Te/Tau]*u(k).
      | Else y(k)=u(k)
      | In case of Reset, the output is initialized to INIT value.
      | In case of permanent reset, y(k)= INIT.
      mask TypeOptions TaskTime: 1ms | 2ms | 5ms | 10ms | 20ms | 50ms | 100ms | 1000ms | SYNC
      mask TypeOptions InType: Tau | Frequency
      mask Display:
      | plot(x,y);
      | plot([min(x),max(x),NaN],[0,0,NaN]);
      | plot(min(-1,min(x)*1.5),min(-1,min(y)*1.5),max(1,max(x)*1.5),max(1,max(y)*1.5));
      | text(min(-0.9,min(x)*1.2),min(-0.9,min(y)*1.2),'First-Order Filter Init');
      | disp(['' TaskTime ''])% ] Cylinders \n Input Size : ' num2str(NTot)])
  Memory : Memory  InheritSampleTime=on
  Product : Product  RndMeth=Zero
  Sum : Sum  Inputs=|+-
  Switch : Switch  Criteria=u2 ~= 0
  rBlowerValveDerivative [%] : Outport  OutputWhenDisabled=reset  InitialOutput=0
      settings: AttributesFormatString=%<OutputWhenDisabled>
  wires:
  [BReset] -> Switch/2
  [tPeriodTask] -> Filtre_1er_ordre_Init/5(PeriodTask [s])
  [tPeriodTask] -> Divide/2
  tPeriodTask [s]/1 -> [tPeriodTask]
  Gain/1 -> Product/2
  Switch/1 -> Product/1  "dErr/dt"
  Product/1 -> Clip/2(In)  "Gain*dErr/dt"
  Constant/1 -> Switch/1
  Sum/1 -> Divide/1
  Max+/1 -> Clip/1(Upper)
  Memory/1 -> Sum/2
  BReset/1 -> [BReset]
  Divide/1 -> Switch/3  "dErr/dt"
  Clip/1(Out) -> rBlowerValveDerivative [%]/1
  [BReset] -> Filtre_1er_ordre_Init/4(RESET)
  Error [mmH2O]/1 -> Filtre_1er_ordre_Init/2(INPUT), Filtre_1er_ordre_Init/3(INIT)
  Min-/1 -> Clip/3(Lower)
  Filtre_1er_ordre_Init/1(OUTPUT) -> Sum/1, Memory/1
  Freq/1 -> Filtre_1er_ordre_Init/1(Frequency [Hz])

== system LIB_CycleControl/Cycle Control/Cycle Control Wrapper/Cycle pController/ValvePosition_Target/Inhalation/Blower Valve Control/PID Blower Valve/Integral Gain/Clip ==
  note: 0,0
  note: 0,0
  note: 0,0
  FreezeUp : Inport
  Upper : Inport  Port=2
  In : Inport  Port=3
  Lower : Inport  Port=4
  FreezeDwn : Inport  Port=5
  Logical Operator : Logic  Operator=NOT  AllPortsSameDT=off  OutDataTypeStr=boolean
  MinMax : MinMax  Inputs=2
  MinMax2 : MinMax  Function=max  Inputs=2
  Multiport Switch : MultiPortSwitch  DataPortOrder=Zero-based contiguous  Inputs=2  zeroidx=on
  Multiport Switch2 : MultiPortSwitch  DataPortOrder=Zero-based contiguous  Inputs=2  zeroidx=on
  Relational Operator : RelationalOperator  Operator=<  RndMeth=Nearest  InputSameDT=on
  Relational Operator1 : RelationalOperator  Operator=>  RndMeth=Nearest  InputSameDT=on
  Switch : Switch  Threshold=1  SaturateOnIntegerOverflow=on  InputSameDT=on
  Switch1 : Switch  Threshold=1  SaturateOnIntegerOverflow=on  InputSameDT=on
  Unit Delay External IC : simulink_need_slupdate/Unit Delay External IC  tsamp=-1
      settings: SourceProductName=Simulink  SourceProductBaseCode=SL
  Unit Delay External IC1 : simulink_need_slupdate/Unit Delay External IC  tsamp=-1
      settings: SourceProductName=Simulink  SourceProductBaseCode=SL
  arround 0.001 : Subsystem
  SatUp : Outport
  Out : Outport  Port=2
  SatDwn : Outport  Port=3
  wires:
  Switch1/1 -> Out/1, [Out]
  Relational Operator1/1 -> Switch1/2, Logical Operator/1
  Switch/1 -> Relational Operator1/1, Switch1/1
  Multiport Switch2/1 -> Switch1/3, Relational Operator1/2
  Relational Operator/1 -> Switch/2, SatUp/1
  In/1 -> arround 0.001/1(In1)
  Logical Operator/1 -> SatDwn/1
  Upper/1 -> Multiport Switch/2, MinMax/1, Unit Delay External IC/2
  Multiport Switch/1 -> Relational Operator/1, Switch/1
  FreezeUp/1 -> Multiport Switch/1
  MinMax/1 -> Multiport Switch/3
  Unit Delay External IC/1 -> MinMax/2
  Lower/1 -> MinMax2/1, Multiport Switch2/2, Unit Delay External IC1/2
  FreezeDwn/1 -> Multiport Switch2/1
  MinMax2/1 -> Multiport Switch2/3
  Unit Delay External IC1/1 -> MinMax2/2
  [Out] -> Unit Delay External IC/1
  [Out] -> Unit Delay External IC1/1
  arround 0.001/1(Out1) -> Relational Operator/2, Switch/3
